simulink subsystem "Motor"  (R2023b)
settings: Solver=VariableStepAuto  StartTime=0.0  StopTime=10.0  RelTol=1e-3
undefined symbols (not defined in the file): DiscIntNeverNeededParam
settings Model: Creator=Usuario_UMA  LastModifiedBy=Usuario_UMA

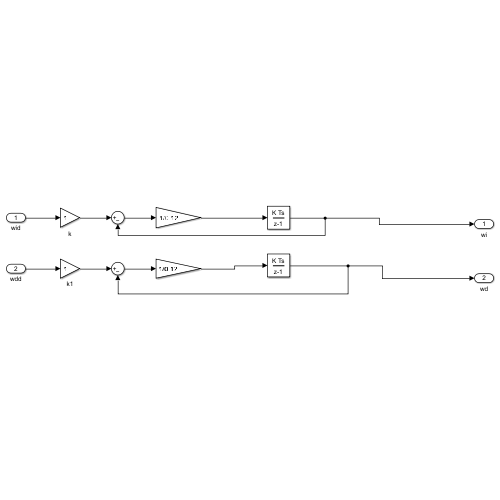
[thumbnail: Simulink's stored preview of the top-level diagram]
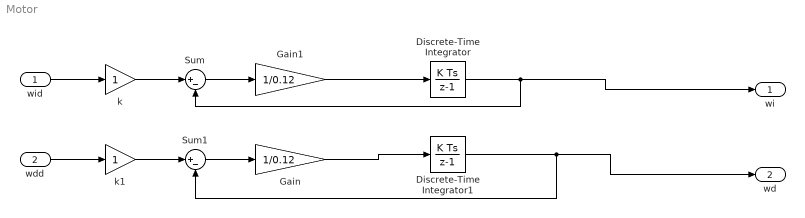
== system Motor ==
  wid : Inport
  wdd : Inport  Port=2
  Discrete-Time Integrator : DiscreteIntegrator  SampleTime=0.025  ICPrevOutput=DiscIntNeverNeededParam  ICPrevScaledInput=DiscIntNeverNeededParam
  Discrete-Time Integrator1 : DiscreteIntegrator  SampleTime=0.025  ICPrevOutput=DiscIntNeverNeededParam  ICPrevScaledInput=DiscIntNeverNeededParam
  Gain : Gain  Gain=1/0.12
  Gain1 : Gain  Gain=1/0.12
  Sum : Sum  Inputs=|+-
  Sum1 : Sum  Inputs=|+-
  k : Gain
  k1 : Gain
  wi : Outport
  wd : Outport  Port=2
  wires:
  wid/1 -> k/1
  k/1 -> Sum/1
  wdd/1 -> k1/1
  k1/1 -> Sum1/1
  Sum/1 -> Gain1/1
  Sum1/1 -> Gain/1
  Gain1/1 -> Discrete-Time Integrator/1
  Discrete-Time Integrator/1 -> Sum/2, wi/1
  Gain/1 -> Discrete-Time Integrator1/1
  Discrete-Time Integrator1/1 -> Sum1/2, wd/1
